simulink model "Slam"  (R2024a)
settings: Solver=VariableStepAuto  StartTime=0.0  StopTime=inf  RelTol=1e-3
undefined symbols (not defined in the file): Angle, Axis
libraries: robotcorelib x3, eeGeneralControl x2
settings Model: Creator=user  LastModifiedBy=quentinlandon

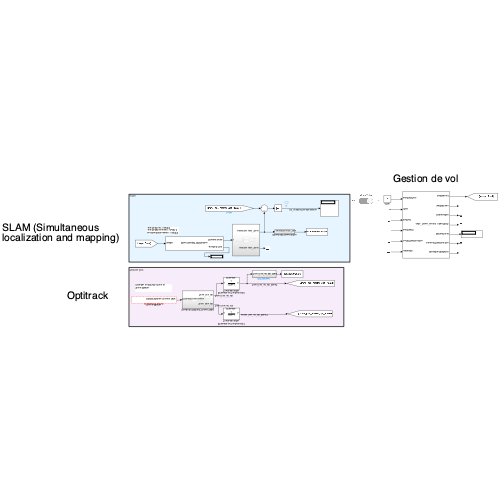
[thumbnail: Simulink's stored preview of the top-level diagram]
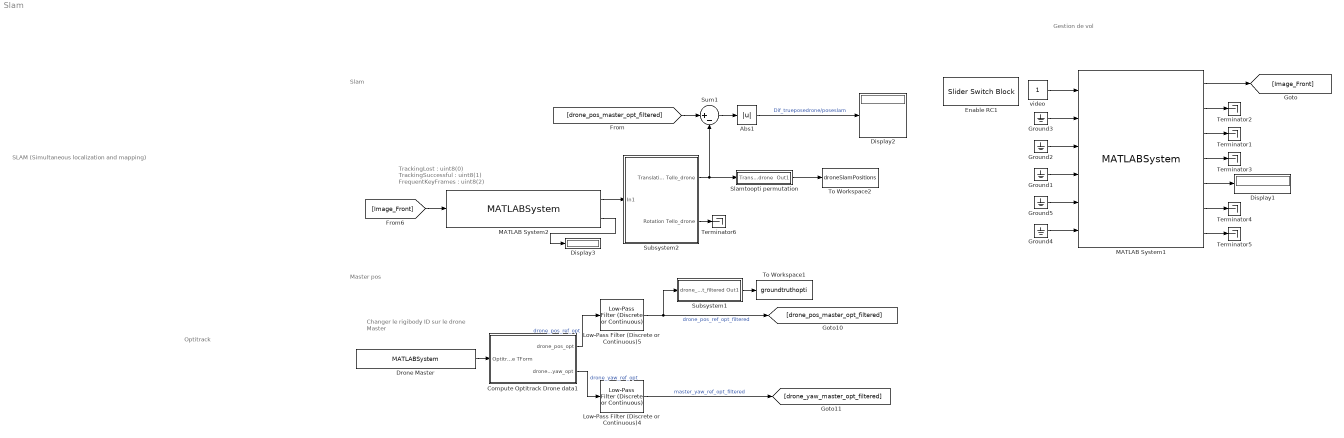
== system Slam ==
  note: Slam
  note: TrackingLost : uint8(0)
      | TrackingSuccessful : uint8(1)
      | FrequentKeyFrames : uint8(2)
  note: Gestion de vol
  note: SLAM (Simultaneous localization and mapping)
  note: Optitrack
  note: Master pos
  note: Changer le rigibody ID sur le drone Master
  Abs1 : Abs  SaturateOnIntegerOverflow=off
  Compute Optitrack Drone data1 : Subsystem
  Display1 : Display
  Display2 : Display
  Display3 : Display
  Drone Master : MATLABSystem  System=OptilinkSystem  HostIP=10.147.125.15  ClientIP=10.147.125.15  RigidbodyID=1  SimulateUsing=Interpreted execution
      mask Type: OptilinkSystem
      mask Display:
      | disp('OptilinkSystem');
      | port_label('output',1,'Drones data');
  Enable RC1 : SliderSwitchBlock
      settings: Values={{'Off', 'On'}, [0 1]}
  Ground{1..5} (5 alike) : Ground
  Low-Pass Filter (Discrete or Continuous)4 : eeGeneralControl/Low-Pass Filter (Discrete or Continuous)  K=1  T=1.5  B=inf  A=-inf  init_option=Inherited from block input  x0=0  Ts=-1
  Low-Pass Filter (Discrete or Continuous)5 : eeGeneralControl/Low-Pass Filter (Discrete or Continuous)  K=1  T=1.5  B=inf  A=-inf  init_option=Inherited from block input  x0=0  Ts=-1
  MATLAB System1 : MATLABSystem  System=Tello_drone_control  droneIP=127.0.0.1  SimulateUsing=Interpreted execution
      mask Type: Tello_drone_control
      mask Display:
      | disp('Tello_drone_control');
      | port_label('input',1,'enableVideo');
      | port_label('input',2,'tkoff');
      | port_label('input',3,'landing');
      | port_label('input',4,'enableRC');
      | port_label('input',5,'cmdVideoDirection');
      | port_label('input',6,'rcspeeds');
      | port_label('output',1,'imageFront');
      | port_label('output',2,'imageDown');
      | port_label('output',3,'Eulerangles');
      | port_label('output',4,'speedXYZ');
      | port_label('output',5,'batteryLevel');
      | port_label('output',6,'currentVideoDirection');
      | port_label('output',7,'hasTakenOffStatus');
  MATLAB System2 : MATLABSystem  System=MonoVisualSLAMSystem  FocalLength=[ 894, 896]  PrincipalPoint=[490,355.6]  ImageSize=[ 720, 960 ]  numPoints=800  numSkipFrames=15  SimulateUsing=Code generation
      mask Type: MonoVisualSLAMSystem
      mask Display:
      | disp('MonoVisualSLAMSystem');
      | port_label('input',1,'Image');
      | port_label('output',1,'Camera Pose');
      | port_label('output',2,'Tracking Lost');
  Slamtoopti permutation : Subsystem
  Subsystem1 : Subsystem
  Subsystem2 : Subsystem
  Sum1 : Sum  Inputs=|+-
  Terminator{1..6} (6 alike) : Terminator
  To Workspace1 : ToWorkspace  VariableName=groundtruthopti  SampleTime=-1
  To Workspace2 : ToWorkspace  VariableName=droneSlamPositions  SampleTime=-1
  video : Constant
  wires:
  [Image_Front] -> MATLAB System2/1
  Slamtoopti permutation/1(Out1) -> To Workspace2/1
  MATLAB System2/2 -> Display3/1
  MATLAB System2/1 -> Subsystem2/1(In1)
  Subsystem2/2(Rotation Tello_drone) -> Terminator6/1
  Subsystem2/1(Translation Tello_drone) -> Slamtoopti permutation/1(Translation Tello_drone), Sum1/2
  Ground3/1 -> MATLAB System1/2
  MATLAB System1/1 -> [Image_Front]
  MATLAB System1/6 -> Terminator4/1
  Ground1/1 -> MATLAB System1/4
  Ground5/1 -> MATLAB System1/5
  MATLAB System1/4 -> Terminator3/1
  MATLAB System1/2 -> Terminator2/1
  MATLAB System1/7 -> Terminator5/1
  video/1 -> MATLAB System1/1
  MATLAB System1/5 -> Display1/1
  Ground2/1 -> MATLAB System1/3
  MATLAB System1/3 -> Terminator1/1
  Ground4/1 -> MATLAB System1/6
  Compute Optitrack Drone data1/2(drone_yaw_opt) -> Low-Pass Filter (Discrete or Continuous)4/1  "drone_yaw_ref_opt"
  Low-Pass Filter (Discrete or Continuous)5/1 -> Subsystem1/1(drone_pos_ref_opt_filtered), [drone_pos_master_opt_filtered]  "drone_pos_ref_opt_filtered"
  Low-Pass Filter (Discrete or Continuous)4/1 -> [drone_yaw_master_opt_filtered]  "master_yaw_ref_opt_filtered"
  Drone Master/1 -> Compute Optitrack Drone data1/1(Optitrack Drone TForm)
  Compute Optitrack Drone data1/1(drone_pos_opt) -> Low-Pass Filter (Discrete or Continuous)5/1  "drone_pos_ref_opt"
  Subsystem1/1(Out1) -> To Workspace1/1
  Sum1/1 -> Abs1/1
  Abs1/1 -> Display2/1  "Dif_trueposedrone/poseslam"
  [drone_pos_master_opt_filtered] -> Sum1/1

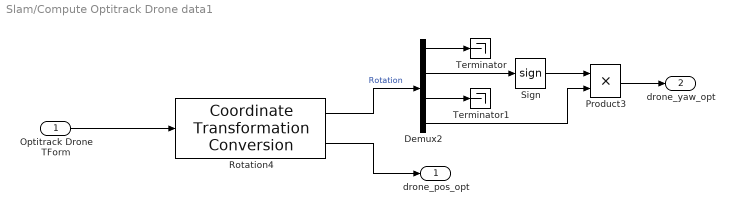
== system Slam/Compute Optitrack Drone data1 ==
  Optitrack Drone TForm : Inport
  Demux2 : Demux
  Product3 : Product
  Rotation4 : robotcorelib/Coordinate Transformation Conversion  InputRepresentation=Homogeneous Transformation  InputEulerSequence=XYZ  ShowTrVecInputPort=on  OutputRepresentation=Axis-Angle  OutputEulerSequence=XYZ  ShowTrVecOutputPort=on  SimulateUsing=Code generation
      settings: LibrarySourceBlock=uavutilslib/Coordinate Transformation Conversion
  Sign : Signum
  Terminator : Terminator
  Terminator1 : Terminator
  drone_pos_opt : Outport
  drone_yaw_opt : Outport  Port=2
  wires:
  Rotation4/2 -> drone_pos_opt/1
  Demux2/4 -> Product3/2
  Rotation4/1 -> Demux2/1  "Rotation"
  Sign/1 -> Product3/1
  Demux2/2 -> Sign/1
  Product3/1 -> drone_yaw_opt/1
  Optitrack Drone TForm/1 -> Rotation4/1
  Demux2/3 -> Terminator1/1
  Demux2/1 -> Terminator/1

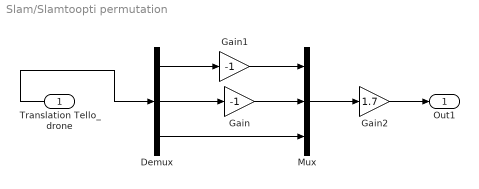
== system Slam/Slamtoopti permutation ==
  Translation Tello_drone : Inport
  Demux : Demux  Outputs=3
  Gain : Gain  Gain=-1
  Gain1 : Gain  Gain=-1
  Gain2 : Gain  Gain=1.7
  Mux : Mux  Inputs=3
  Out1 : Outport
  wires:
  Demux/2 -> Gain/1
  Demux/1 -> Gain1/1
  Mux/1 -> Gain2/1
  Gain/1 -> Mux/2
  Demux/3 -> Mux/3
  Gain1/1 -> Mux/1
  Gain2/1 -> Out1/1
  Translation Tello_drone/1 -> Demux/1

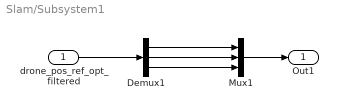
== system Slam/Subsystem1 ==
  drone_pos_ref_opt_filtered : Inport
  Demux1 : Demux  Outputs=3
  Mux1 : Mux  Inputs=3
  Out1 : Outport
  wires:
  drone_pos_ref_opt_filtered/1 -> Demux1/1
  Mux1/1 -> Out1/1
  Demux1/3 -> Mux1/3
  Demux1/2 -> Mux1/2
  Demux1/1 -> Mux1/1

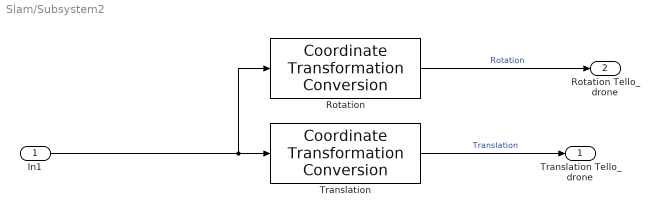
== system Slam/Subsystem2 ==
  In1 : Inport
  Rotation : robotcorelib/Coordinate Transformation Conversion  InputRepresentation=Homogeneous Transformation  InputEulerSequence=ZYX  ShowTrVecInputPort=on  OutputRepresentation=Rotation Matrix  OutputEulerSequence=ZYX  ShowTrVecOutputPort=off  SimulateUsing=Code generation
      settings: LibrarySourceBlock=uavutilslib/Coordinate Transformation Conversion
  Translation : robotcorelib/Coordinate Transformation Conversion  InputRepresentation=Homogeneous Transformation  InputEulerSequence=ZYX  ShowTrVecInputPort=on  OutputRepresentation=Translation Vector  OutputEulerSequence=ZYX  ShowTrVecOutputPort=on  SimulateUsing=Code generation
      settings: LibrarySourceBlock=uavutilslib/Coordinate Transformation Conversion
  Translation Tello_drone : Outport
  Rotation Tello_drone : Outport  Port=2
  wires:
  Translation/1 -> Translation Tello_drone/1  "Translation"
  Rotation/1 -> Rotation Tello_drone/1  "Rotation"
  In1/1 -> Rotation/1, Translation/1
